simulink model "myrobot"  (R2021a)
settings: Solver=VariableStepAuto  StartTime=0.0  StopTime=10.0  RelTol=1e-3
libraries: simulink x1
settings Model: Creator=duong  LastModifiedBy=duong

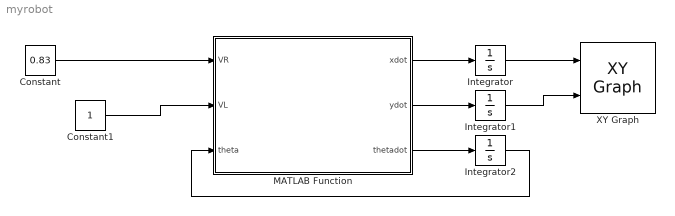
== system myrobot ==
  Constant : Constant  Value=0.83
  Constant1 : Constant
  Integrator : Integrator
  Integrator1 : Integrator
  Integrator2 : Integrator
  MATLAB Function : MATLAB Function  TreatAsAtomicUnit=on
  XY Graph : simulink/Sinks/XY Graph  xmin=-2  xmax=2  ymin=-2  ymax=2  st=-1
  wires:
  MATLAB Function/3(thetadot) -> Integrator2/1
  Integrator2/1 -> MATLAB Function/3(theta)
  MATLAB Function/1(xdot) -> Integrator/1
  MATLAB Function/2(ydot) -> Integrator1/1
  Integrator/1 -> XY Graph/1
  Integrator1/1 -> XY Graph/2
  Constant/1 -> MATLAB Function/1(VR)
  Constant1/1 -> MATLAB Function/2(VL)

== matlab function myrobot/MATLAB Function ==
  data: VR input; xdot output; VL input; theta input; ydot output; thetadot output
function [xdot, ydot, thetadot] = fcn(VR, VL,theta)

l=0.18; % distance between 2 driven wheels
xdot=(VR+VL)/2*cos(theta);
ydot=(VR+VL)/2*sin(theta);
thetadot=(VR-VL)/l;
